simulink model "DPendulum_Simulink"  (R2023a)
settings: Solver=VariableStepAuto  StartTime=0.0  StopTime=5  RelTol=1e-3
libraries: slpidlib x1
settings Model: Creator=Inovicht  LastModifiedBy=Inovicht

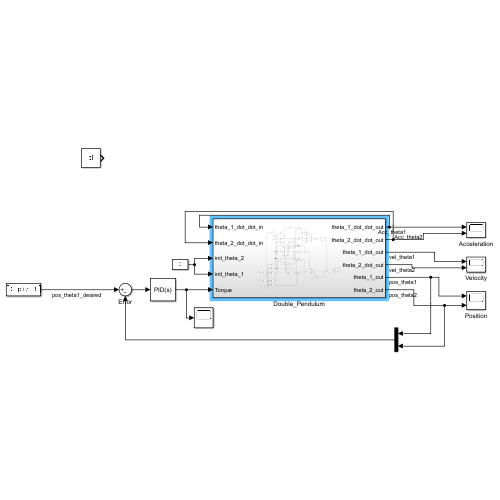
[thumbnail: Simulink's stored preview of the top-level diagram]
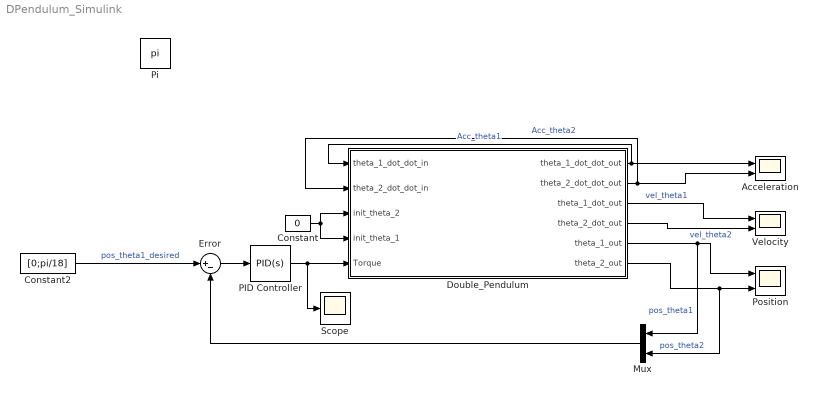
== system DPendulum_Simulink ==
  Acceleration : Scope  NumInputPorts=2
  Constant : Constant  Value=0
  Constant2 : Constant  Value=[0;pi/18]
  Double_Pendulum : Subsystem
  Error : Sum  Inputs=|+-
  Mux : Mux  Inputs=2
  PID Controller : slpidlib/PID Controller  Controller=PID  Form=Parallel  TimeDomain=Continuous-time  UseExternalTs=off  SampleTime=-1  IntegratorMethod=Forward Euler  FilterMethod=Forward Euler  ControllerParametersSource=internal  P=20  I=0  UseKiTs=off  D=0  N=100  UseFilter=on  TunerSelectOption=Transfer Function Based (PID Tuner App)  InitialConditionSource=internal  InitialConditionForIntegrator=0  InitialConditionForFilter=0  DifferentiatorICPrevScaledInput=0  ExternalReset=none  TrackingMode=off  Kt=1  LimitOutput=off  SatLimitsSource=internal  UpperSaturationLimit=inf  LowerSaturationLimit=-inf  LinearizeAsGain=on  AntiWindupMode=none  Kb=1  LimitIntegrator=off  UpperIntegratorSaturationLimit=inf  LowerIntegratorSaturationLimit=-inf  POutMin=[]  POutMax=[]  IOutMin=[]  IOutMax=[]  DOutMin=[]  DOutMax=[]  NOutMin=[]  NOutMax=[]  SumOutMin=[]  SumOutMax=[]  SaturationOutMin=[]  SaturationOutMax=[]  PParamMin=[]  PParamMax=[]  IParamMin=[]  IParamMax=[]  DParamMin=[]  DParamMax=[]  NParamMin=[]  NParamMax=[]  KbParamMin=[]  KbParamMax=[]  KtParamMin=[]  KtParamMax=[]  KbOutMin=[]  KbOutMax=[]  KtOutMin=[]  KtOutMax=[]  IntegratorOutMin=[]  IntegratorOutMax=[]  FilterOutMin=[]  FilterOutMax=[]  SumI1OutMin=[]  SumI1OutMax=[]  SumI2OutMin=[]  SumI2OutMax=[]  SumI3OutMin=[]  SumI3OutMax=[]  SumI4OutMin=[]  SumI4OutMax=[]  SumDOutMin=[]  SumDOutMax=[]  DifferentiatorOutMin=[]  DifferentiatorOutMax=[]  FilterDiffOutCoefMin=[]  FilterDiffOutCoefMax=[]  ReciprocalOutMin=[]  ReciprocalOutMax=[]  SumDenOutMin=[]  SumDenOutMax=[]  SumNumOutMin=[]  SumNumOutMax=[]  DivideOutMin=[]  DivideOutMax=[]  UdiffTsProdOutMin=[]  UdiffTsProdOutMax=[]  NTsProdOutMin=[]  NTsProdOutMax=[]  UintegralTsProdOutMin=[]  UintegralTsProdOutMax=[]  UngainTsProdOutMin=[]  UngainTsProdOutMax=[]  ClampingZeroOutDataTypeStr=Inherit: Inherit via back propagation  ClampingZeroOutMin=[]  ClampingZeroOutMax=[]  FilterDenConstantOutDataTypeStr=Inherit: Inherit via back propagation  FilterDenConstantOutMin=[]  FilterDenConstantOutMax=[]  PCopyOutDataTypeStr=Inherit: Inherit via back propagation  PCopyOutMin=[]  PCopyOutMax=[]  NCopyOutDataTypeStr=Inherit: Inherit via back propagation  NCopyOutMin=[]  NCopyOutMax=[]  IntegratorContinuousStateAttributes=''  IntegratorStateMustResolveToSignalObject=off  IntegratorRTWStateStorageClass=Auto  FilterContinuousStateAttributes=''  FilterStateMustResolveToSignalObject=off  FilterRTWStateStorageClass=Auto  ParallelPVariant=InternalParameters  IdealPVariant=Disabled  IVariant=InternalParameters  DVariant=InternalParameters  IntegratorVariant=Continuous  SatVariant=Disabled  AWVariant=Passthrough  PCopyVariant=Disabled  TRVariant=Disabled  FdbkBlocksVariant=Forward  IdealPFdbkVariant=Disabled  SatFdbkVariant=Disabled  DerivativeFilterVariant=ContFilter  NVariant=InternalParameters  NCopyVariant=Disabled  FilterICVariant=InternalICsFilter  IntegratorICVariant=InternalICs  ExternalResetVariant=Disabled  TRSumVariant=Passthrough  SumFdbkVariant=Disabled  SumVariant=Sum_PID  TsampFilterVariant=InternalTs  TsampNgainVariant=Passthrough  TsampIntegralVariant=Disabled_SignalSpec  ExternalSaturationOutDataTypeStr=Inherit: Same as second input
  Pi : Constant  Value=pi  OutDataTypeStr=Inherit: Inherit via back propagation
  Position : Scope  NumInputPorts=2
  Scope : Scope
  Velocity : Scope  NumInputPorts=2
  wires:
  Constant/1 -> Double_Pendulum/4(init_theta_1), Double_Pendulum/3(init_theta_2)
  Double_Pendulum/5(theta_1_out) -> Mux/1, Position/1  "pos_theta1"
  Double_Pendulum/1(theta_1_dot_dot_out) -> Acceleration/1, Double_Pendulum/1(theta_1_dot_dot_in)  "Acc_theta1"
  Double_Pendulum/6(theta_2_out) -> Mux/2, Position/2  "pos_theta2"
  Double_Pendulum/2(theta_2_dot_dot_out) -> Double_Pendulum/2(theta_2_dot_dot_in), Acceleration/2  "Acc_theta2"
  Double_Pendulum/3(theta_1_dot_out) -> Velocity/1  "vel_theta1"
  Double_Pendulum/4(theta_2_dot_out) -> Velocity/2  "vel_theta2"
  Constant2/1 -> Error/1  "pos_theta1_desired"
  Mux/1 -> Error/2
  Error/1 -> PID Controller/1
  PID Controller/1 -> Scope/1, Double_Pendulum/5(Torque)

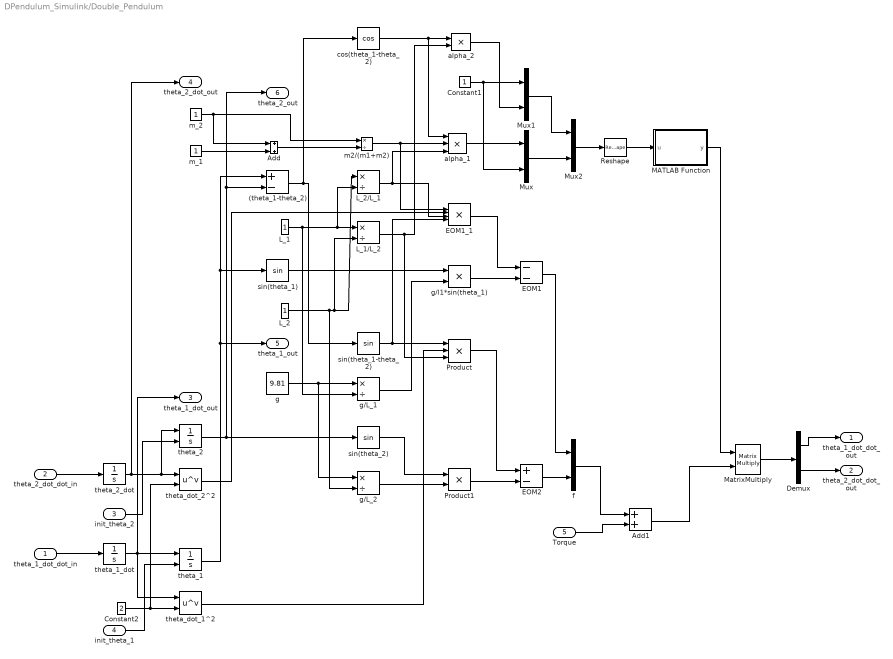
== system DPendulum_Simulink/Double_Pendulum ==
  theta_1_dot_dot_in : Inport
  theta_2_dot_dot_in : Inport  Port=2
  init_theta_2 : Inport  Port=3
  init_theta_1 : Inport  Port=4
  Torque : Inport  Port=5
  (theta_1-theta_2) : Sum  Inputs=+-
  Add : Sum
  Add1 : Sum
  Constant1 : Constant
  Constant2 : Constant  Value=2
  Demux : Demux  Outputs=2
  EOM1 : Sum  Inputs=--
  EOM1_1 : Product  Inputs=4
  EOM2 : Sum  Inputs=+-
  L_1 : Constant
  L_1/L_2 : Product  Inputs=*/
  L_2 : Constant
  L_2/L_1 : Product  Inputs=*/
  MATLAB Function : MATLAB Function  TreatAsAtomicUnit=on
  MatrixMultiply : Product  Multiplication=Matrix(*)
  Mux : Mux  Inputs=2
  Mux1 : Mux  Inputs=2
  Mux2 : Mux  Inputs=2
  Product : Product  Inputs=3
  Product1 : Product
  Reshape : Reshape  OutputDimensionality=Customize  OutputDimensions=[2,2]
  alpha_1 : Product  Inputs=3
  alpha_2 : Product
  cos(theta_1-theta_2) : Trigonometry  Operator=cos
  f : Mux  Inputs=2
  g : Constant  Value=9.81
  g/L_1 : Product  Inputs=*/
  g/L_2 : Product  Inputs=*/
  g/l1*sin(theta_1) : Product
  m2/(m1+m2) : Product  Inputs=*/
  m_1 : Constant
  m_2 : Constant
  sin(theta_1) : Trigonometry
  sin(theta_1-theta_2) : Trigonometry
  sin(theta_2) : Trigonometry
  theta_1 : Integrator  InitialConditionSource=external  InitialCondition=pi/4
  theta_1_dot : Integrator
  theta_2 : Integrator  InitialConditionSource=external  InitialCondition=pi/4
  theta_2_dot : Integrator
  theta_dot_1^2 : Math  Operator=pow
  theta_dot_2^2 : Math  Operator=pow
  theta_1_dot_dot_out : Outport
  theta_2_dot_dot_out : Outport  Port=2
  theta_1_dot_out : Outport  Port=3
  theta_2_dot_out : Outport  Port=4
  theta_1_out : Outport  Port=5
  theta_2_out : Outport  Port=6
  wires:
  theta_1_dot_dot_in/1 -> theta_1_dot/1
  Product1/1 -> EOM2/2
  theta_2_dot_dot_in/1 -> theta_2_dot/1
  Product/1 -> EOM2/1
  theta_2_dot/1 -> theta_dot_2^2/1, theta_2/1, theta_2_dot_out/1
  init_theta_1/1 -> theta_1/2
  alpha_1/1 -> Mux/1
  init_theta_2/1 -> theta_2/2
  L_1/L_2/1 -> alpha_2/2, Product/3
  theta_1/1 -> (theta_1-theta_2)/1, sin(theta_1)/1, theta_1_out/1
  theta_1_dot/1 -> theta_dot_1^2/1, theta_1/1, theta_1_dot_out/1
  Constant2/1 -> theta_dot_1^2/2, theta_dot_2^2/2
  m_2/1 -> m2/(m1+m2)/1, Add/1
  m_1/1 -> Add/2
  Constant1/1 -> Mux/2, Mux1/1
  alpha_2/1 -> Mux1/2
  theta_2/1 -> (theta_1-theta_2)/2, theta_2_out/1, sin(theta_2)/1
  theta_dot_2^2/1 -> EOM1_1/2
  theta_dot_1^2/1 -> Product/2
  EOM1/1 -> f/1
  Add/1 -> m2/(m1+m2)/2
  L_2/1 -> L_1/L_2/2, L_2/L_1/1, g/L_2/2
  (theta_1-theta_2)/1 -> sin(theta_1-theta_2)/1, cos(theta_1-theta_2)/1
  MATLAB Function/1(y) -> MatrixMultiply/1
  L_1/1 -> L_2/L_1/2, L_1/L_2/1, g/L_1/2
  sin(theta_1)/1 -> g/l1*sin(theta_1)/1
  g/1 -> g/L_2/1, g/L_1/1
  m2/(m1+m2)/1 -> alpha_1/2, EOM1_1/1
  cos(theta_1-theta_2)/1 -> alpha_1/1, alpha_2/1
  EOM2/1 -> f/2
  L_2/L_1/1 -> EOM1_1/3, alpha_1/3
  sin(theta_1-theta_2)/1 -> EOM1_1/4, Product/1
  Mux/1 -> Mux2/2
  g/L_1/1 -> g/l1*sin(theta_1)/2
  g/l1*sin(theta_1)/1 -> EOM1/2
  sin(theta_2)/1 -> Product1/1
  g/L_2/1 -> Product1/2
  Demux/1 -> theta_1_dot_dot_out/1
  EOM1_1/1 -> EOM1/1
  Mux1/1 -> Mux2/1
  Mux2/1 -> Reshape/1
  f/1 -> Add1/1
  Reshape/1 -> MATLAB Function/1(u)
  MatrixMultiply/1 -> Demux/1
  Demux/2 -> theta_2_dot_dot_out/1
  Torque/1 -> Add1/2
  Add1/1 -> MatrixMultiply/2

== matlab function DPendulum_Simulink/Double_Pendulum/MATLAB Function ==
  data: u input; y output
function y = inverse_2x2(u)
    % u is a 2x2 matrix
    y = inv(u);
end
